simulink library "PMSM_Library"  (R2023a)
settings: Solver=VariableStepAuto  StartTime=0.0  StopTime=10.0  RelTol=1e-3  EnableMultiTasking=on
settings Model: Creator=michaelsun  LastModifiedBy=洲
settings SolverCC: AlgebraicLoopSolver=TrustRegion
settings DataIOCC: LimitDataPoints=on
settings OptimizationCC: LifeSpan=inf
settings DebuggingCC: UnconnectedInputMsg=warning  UnconnectedOutputMsg=warning  UnconnectedLineMsg=warning  AllowSymbolicDim=off  SFUnexpectedBacktrackingDiag=warning  SFNoUnconditionalDefaultTransitionDiag=warning  SFExecutionAtInitializationDiag=none  ArithmeticOperatorsInVariantConditions=warning
settings ModelReferenceCC: EnableRefExpFcnMdlSchedulingChecks=on  PropagateSignalLabelsOutOfModel=off
settings SFSimCC: SimUseLocalCustomCode=off  CustomCodeUndefinedFunction=UseInterfaceOnly
settings RTWCC: RTWUseLocalCustomCode=off  DLArmComputeVersion=19.05
settings CodeAppCC: StateflowObjectComments=on
settings GRTTargetCC: TargetLangStandard=C89/C90 (ANSI)
settings ConfigComp: CovMetricSettings=dw  CovSaveCumulativeToWorkspaceVar=on  CovSaveSingleToWorkspaceVar=on  CovExternalEMLEnable=off

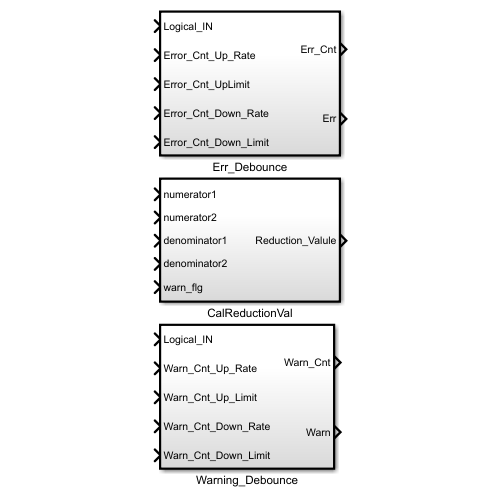
[thumbnail: Simulink's stored preview of the top-level diagram]
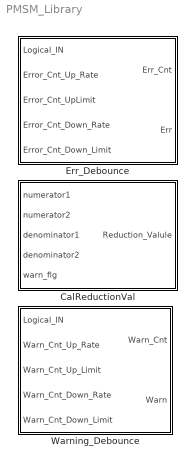
== system PMSM_Library ==
  CalReductionVal : Subsystem  TreatAsAtomicUnit=on  RTWFcnName=CalReductionVal  RTWFileName=CalReductionVal
      settings: RTWSystemCode=Inline  RTWFcnNameOpts=User specified  RTWFileNameOpts=User specified
  Err_Debounce : Subsystem  TreatAsAtomicUnit=on  RTWFcnName=Err_Debounce  RTWFileName=Err_Debounce
      settings: RTWSystemCode=Inline  RTWFcnNameOpts=User specified  RTWFileNameOpts=User specified
  Warning_Debounce : Subsystem  TreatAsAtomicUnit=on  RTWFcnName=Warning_Debounce  RTWFileName=Warning_Debounce
      settings: RTWSystemCode=Inline  RTWFcnNameOpts=User specified  RTWFileNameOpts=User specified

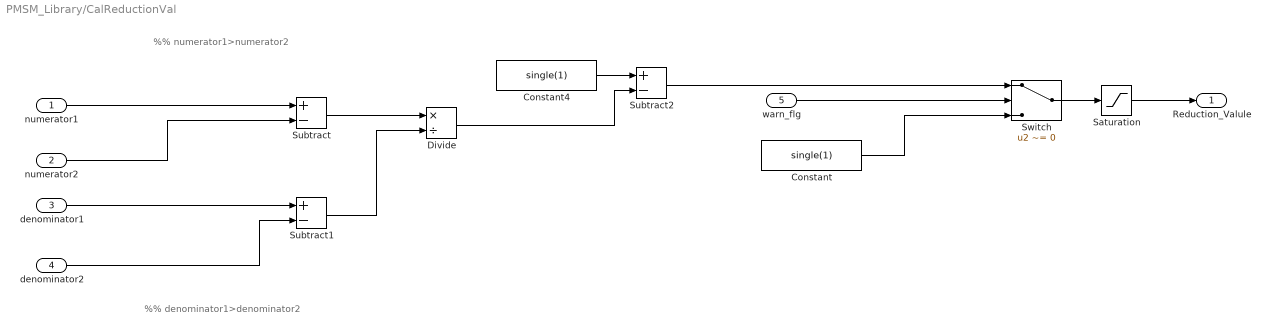
== system PMSM_Library/CalReductionVal ==
  note: %% numerator1>numerator2
  note: %% denominator1>denominator2
  numerator1 : Inport
  numerator2 : Inport  Port=2
  denominator1 : Inport  Port=3
  denominator2 : Inport  Port=4
  warn_flg : Inport  Port=5
  Constant : Constant  Value=single(1)
  Constant4 : Constant  Value=single(1)
  Divide : Product  Inputs=*/
  Saturation : Saturate  UpperLimit=1.0  LowerLimit=0.0
  Subtract : Sum  Inputs=+-
  Subtract1 : Sum  Inputs=+-
  Subtract2 : Sum  Inputs=+-
  Switch : Switch  Criteria=u2 ~= 0  SaturateOnIntegerOverflow=off  InputSameDT=off
  Reduction_Valule : Outport
  wires:
  Saturation/1 -> Reduction_Valule/1
  numerator2/1 -> Subtract/2
  denominator1/1 -> Subtract1/1
  denominator2/1 -> Subtract1/2
  Constant4/1 -> Subtract2/1
  Constant/1 -> Switch/3
  warn_flg/1 -> Switch/2
  Switch/1 -> Saturation/1
  Subtract2/1 -> Switch/1
  Divide/1 -> Subtract2/2
  Subtract1/1 -> Divide/2
  Subtract/1 -> Divide/1
  numerator1/1 -> Subtract/1

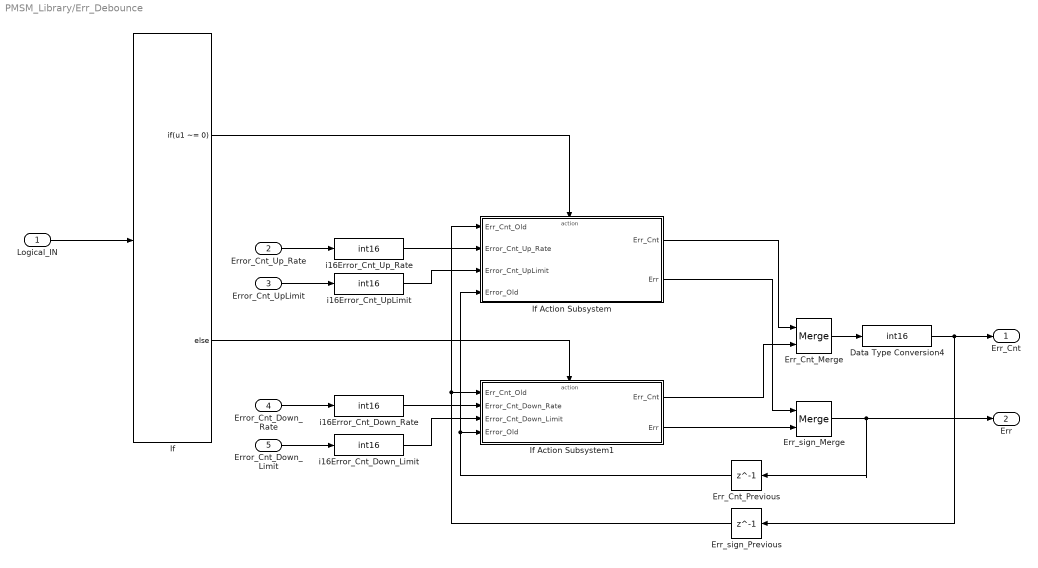
== system PMSM_Library/Err_Debounce ==
  Logical_IN : Inport
  Error_Cnt_Up_Rate : Inport  Port=2
  Error_Cnt_UpLimit : Inport  Port=3
  Error_Cnt_Down_Rate : Inport  Port=4
  Error_Cnt_Down_Limit : Inport  Port=5
  Data Type Conversion4 : DataTypeConversion  OutDataTypeStr=int16  SaturateOnIntegerOverflow=off  RndMeth=Floor
  Err_Cnt_Merge : Merge
  Err_Cnt_Previous : Delay  DelayLength=1  InitialCondition=boolean(0)
  Err_sign_Merge : Merge
  Err_sign_Previous : Delay  DelayLength=1
  If : If  IfExpression=u1 ~= 0
  If Action Subsystem : Subsystem  TreatAsAtomicUnit=on
  If Action Subsystem1 : Subsystem  TreatAsAtomicUnit=on
  i16Error_Cnt_Down_Limit : DataTypeConversion  OutDataTypeStr=int16  SaturateOnIntegerOverflow=off  RndMeth=Floor
  i16Error_Cnt_Down_Rate : DataTypeConversion  OutDataTypeStr=int16  SaturateOnIntegerOverflow=off  RndMeth=Floor
  i16Error_Cnt_UpLimit : DataTypeConversion  OutDataTypeStr=int16  SaturateOnIntegerOverflow=off  RndMeth=Floor
  i16Error_Cnt_Up_Rate : DataTypeConversion  OutDataTypeStr=int16  SaturateOnIntegerOverflow=off  RndMeth=Floor
  Err_Cnt : Outport
  Err : Outport  Port=2
  wires:
  Data Type Conversion4/1 -> Err_sign_Previous/1, Err_Cnt/1
  i16Error_Cnt_Up_Rate/1 -> If Action Subsystem/2(Error_Cnt_Up_Rate)
  i16Error_Cnt_UpLimit/1 -> If Action Subsystem/3(Error_Cnt_UpLimit)
  i16Error_Cnt_Down_Rate/1 -> If Action Subsystem1/2(Error_Cnt_Down_Rate)
  i16Error_Cnt_Down_Limit/1 -> If Action Subsystem1/3(Error_Cnt_Down_Limit)
  Err_Cnt_Previous/1 -> If Action Subsystem/4(Error_Old), If Action Subsystem1/4(Error_Old)
  Err_sign_Merge/1 -> Err/1, Err_Cnt_Previous/1
  If Action Subsystem/2(Err) -> Err_sign_Merge/1
  If Action Subsystem1/2(Err) -> Err_sign_Merge/2
  Error_Cnt_Down_Limit/1 -> i16Error_Cnt_Down_Limit/1
  Error_Cnt_Up_Rate/1 -> i16Error_Cnt_Up_Rate/1
  Error_Cnt_Down_Rate/1 -> i16Error_Cnt_Down_Rate/1
  Logical_IN/1 -> If/1
  Error_Cnt_UpLimit/1 -> i16Error_Cnt_UpLimit/1
  If Action Subsystem1/1(Err_Cnt) -> Err_Cnt_Merge/2
  If Action Subsystem/1(Err_Cnt) -> Err_Cnt_Merge/1
  If/2 -> If Action Subsystem1/Action
  If/1 -> If Action Subsystem/Action
  Err_sign_Previous/1 -> If Action Subsystem1/1(Err_Cnt_Old), If Action Subsystem/1(Err_Cnt_Old)
  Err_Cnt_Merge/1 -> Data Type Conversion4/1

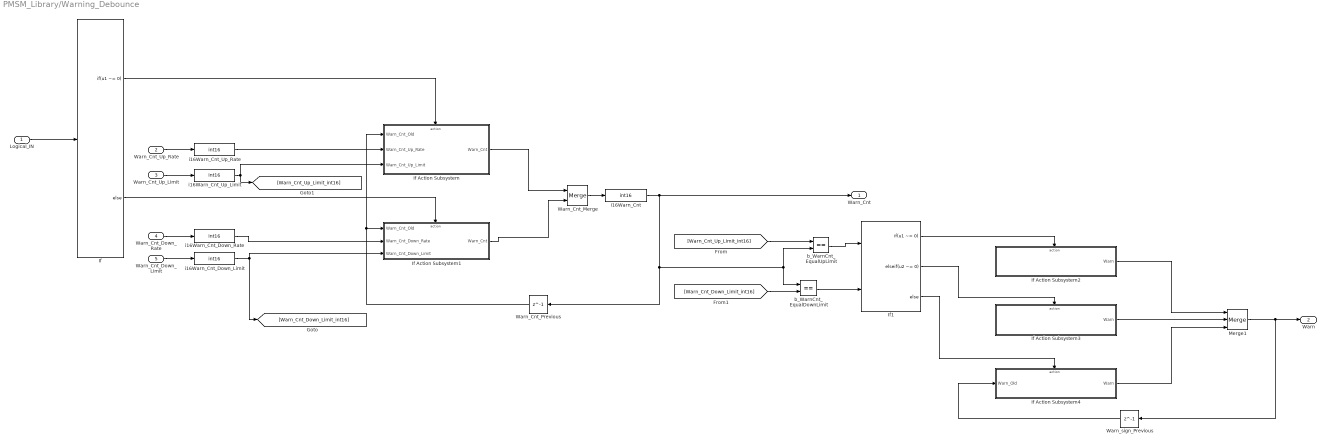
== system PMSM_Library/Warning_Debounce ==
  Logical_IN : Inport
  Warn_Cnt_Up_Rate : Inport  Port=2
  Warn_Cnt_Up_Limit : Inport  Port=3
  Warn_Cnt_Down_Rate : Inport  Port=4
  Warn_Cnt_Down_Limit : Inport  Port=5
  If : If  IfExpression=u1 ~= 0
  If Action Subsystem : Subsystem  TreatAsAtomicUnit=on
  If Action Subsystem1 : Subsystem  TreatAsAtomicUnit=on
  If Action Subsystem2 : Subsystem  TreatAsAtomicUnit=on
  If Action Subsystem3 : Subsystem  TreatAsAtomicUnit=on
  If Action Subsystem4 : Subsystem  TreatAsAtomicUnit=on
  If1 : If  NumInputs=2  IfExpression=u1 ~= 0  ElseIfExpressions=u2 ~= 0
  Merge1 : Merge  Inputs=3
  Warn_Cnt_Merge : Merge
  Warn_Cnt_Previous : Delay  DelayLength=1
  Warn_sign_Previous : Delay  DelayLength=1
  b_WarnCnt_EqualDownLimit : RelationalOperator  Operator===  OutDataTypeStr=boolean  InputSameDT=off
  b_WarnCnt_EqualUpLimit : RelationalOperator  Operator===  OutDataTypeStr=boolean  InputSameDT=off
  i16Warn_Cnt : DataTypeConversion  OutDataTypeStr=int16  SaturateOnIntegerOverflow=off  RndMeth=Floor
  i16Warn_Cnt_Down_Limit : DataTypeConversion  OutDataTypeStr=int16  SaturateOnIntegerOverflow=off  RndMeth=Floor
  i16Warn_Cnt_Down_Rate : DataTypeConversion  OutDataTypeStr=int16  SaturateOnIntegerOverflow=off  RndMeth=Floor
  i16Warn_Cnt_Up_Limit : DataTypeConversion  OutDataTypeStr=int16  SaturateOnIntegerOverflow=off  RndMeth=Floor
  i16Warn_Cnt_Up_Rate : DataTypeConversion  OutDataTypeStr=int16  SaturateOnIntegerOverflow=off  RndMeth=Floor
  Warn_Cnt : Outport
  Warn : Outport  Port=2
  wires:
  Warn_sign_Previous/1 -> If Action Subsystem4/1(Warn_Old)
  Merge1/1 -> Warn/1, Warn_sign_Previous/1
  If Action Subsystem4/1(Warn) -> Merge1/3
  If Action Subsystem2/1(Warn) -> Merge1/1
  If Action Subsystem3/1(Warn) -> Merge1/2
  If1/3 -> If Action Subsystem4/Action
  If1/2 -> If Action Subsystem3/Action
  If1/1 -> If Action Subsystem2/Action
  b_WarnCnt_EqualDownLimit/1 -> If1/2
  b_WarnCnt_EqualUpLimit/1 -> If1/1
  [Warn_Cnt_Down_Limit_int16] -> b_WarnCnt_EqualDownLimit/2
  [Warn_Cnt_Up_Limit_int16] -> b_WarnCnt_EqualUpLimit/1
  Warn_Cnt_Merge/1 -> i16Warn_Cnt/1
  Warn_Cnt_Previous/1 -> If Action Subsystem/1(Warn_Cnt_Old), If Action Subsystem1/1(Warn_Cnt_Old)
  If/1 -> If Action Subsystem/Action
  If/2 -> If Action Subsystem1/Action
  If Action Subsystem/1(Warn_Cnt) -> Warn_Cnt_Merge/1
  If Action Subsystem1/1(Warn_Cnt) -> Warn_Cnt_Merge/2
  Warn_Cnt_Up_Limit/1 -> i16Warn_Cnt_Up_Limit/1
  Logical_IN/1 -> If/1
  Warn_Cnt_Down_Rate/1 -> i16Warn_Cnt_Down_Rate/1
  Warn_Cnt_Up_Rate/1 -> i16Warn_Cnt_Up_Rate/1
  Warn_Cnt_Down_Limit/1 -> i16Warn_Cnt_Down_Limit/1
  i16Warn_Cnt_Down_Limit/1 -> If Action Subsystem1/3(Warn_Cnt_Down_Limit), [Warn_Cnt_Down_Limit_int16]
  i16Warn_Cnt_Down_Rate/1 -> If Action Subsystem1/2(Warn_Cnt_Down_Rate)
  i16Warn_Cnt_Up_Limit/1 -> [Warn_Cnt_Up_Limit_int16], If Action Subsystem/3(Warn_Cnt_Up_Limit)
  i16Warn_Cnt_Up_Rate/1 -> If Action Subsystem/2(Warn_Cnt_Up_Rate)
  i16Warn_Cnt/1 -> Warn_Cnt/1, Warn_Cnt_Previous/1, b_WarnCnt_EqualUpLimit/2, b_WarnCnt_EqualDownLimit/1

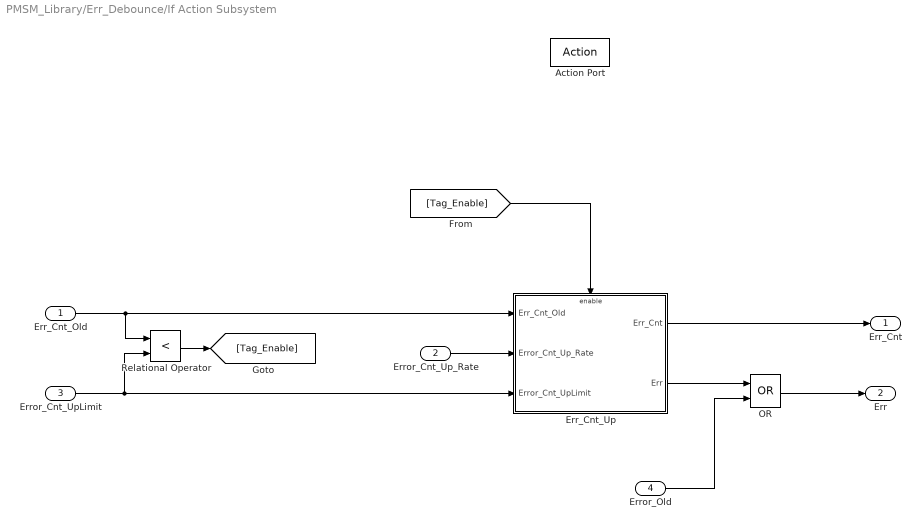
== system PMSM_Library/Err_Debounce/If Action Subsystem ==
  Err_Cnt_Old : Inport
  Error_Cnt_Up_Rate : Inport  Port=2
  Error_Cnt_UpLimit : Inport  Port=3
  Error_Old : Inport  Port=4
  Action Port : ActionPort
  Err_Cnt_Up : Subsystem  RTWFcnName=Err_Cnt_Up
      settings: RTWSystemCode=Inline  RTWFcnNameOpts=User specified
  OR : Logic  Operator=OR  AllPortsSameDT=off  OutDataTypeStr=boolean
  Relational Operator : RelationalOperator  Operator=<  OutDataTypeStr=boolean  InputSameDT=off
  Err_Cnt : Outport
  Err : Outport  Port=2
  wires:
  [Tag_Enable] -> Err_Cnt_Up/Enable
  Relational Operator/1 -> [Tag_Enable]
  Err_Cnt_Up/2(Err) -> OR/1
  Err_Cnt_Up/1(Err_Cnt) -> Err_Cnt/1
  Error_Cnt_UpLimit/1 -> Relational Operator/2, Err_Cnt_Up/3(Error_Cnt_UpLimit)
  Error_Cnt_Up_Rate/1 -> Err_Cnt_Up/2(Error_Cnt_Up_Rate)
  Err_Cnt_Old/1 -> Err_Cnt_Up/1(Err_Cnt_Old), Relational Operator/1
  Error_Old/1 -> OR/2
  OR/1 -> Err/1

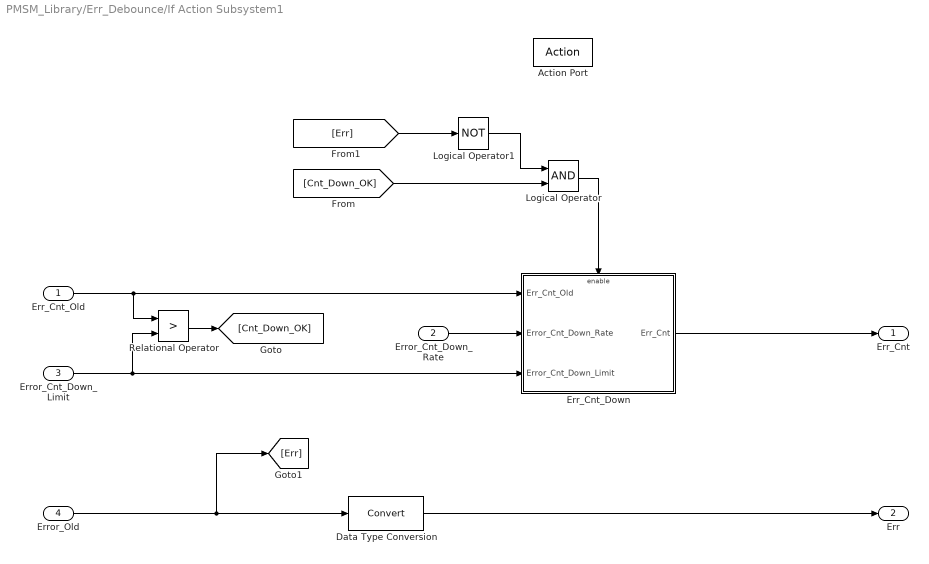
== system PMSM_Library/Err_Debounce/If Action Subsystem1 ==
  Err_Cnt_Old : Inport
  Error_Cnt_Down_Rate : Inport  Port=2
  Error_Cnt_Down_Limit : Inport  Port=3
  Error_Old : Inport  Port=4
  Action Port : ActionPort
  Data Type Conversion : DataTypeConversion  SaturateOnIntegerOverflow=off  RndMeth=Floor
  Err_Cnt_Down : Subsystem  RTWFcnName=Err_Cnt_Down
      settings: RTWSystemCode=Inline  RTWFcnNameOpts=User specified
  Logical Operator : Logic  AllPortsSameDT=off  OutDataTypeStr=boolean
  Logical Operator1 : Logic  Operator=NOT  AllPortsSameDT=off  OutDataTypeStr=boolean
  Relational Operator : RelationalOperator  Operator=>  OutDataTypeStr=boolean  InputSameDT=off
  Err_Cnt : Outport
  Err : Outport  Port=2
  wires:
  Data Type Conversion/1 -> Err/1
  Error_Old/1 -> Data Type Conversion/1, [Err]
  Logical Operator1/1 -> Logical Operator/1
  [Err] -> Logical Operator1/1
  Logical Operator/1 -> Err_Cnt_Down/Enable
  [Cnt_Down_OK] -> Logical Operator/2
  Error_Cnt_Down_Rate/1 -> Err_Cnt_Down/2(Error_Cnt_Down_Rate)
  Relational Operator/1 -> [Cnt_Down_OK]
  Err_Cnt_Down/1(Err_Cnt) -> Err_Cnt/1
  Error_Cnt_Down_Limit/1 -> Relational Operator/2, Err_Cnt_Down/3(Error_Cnt_Down_Limit)
  Err_Cnt_Old/1 -> Err_Cnt_Down/1(Err_Cnt_Old), Relational Operator/1

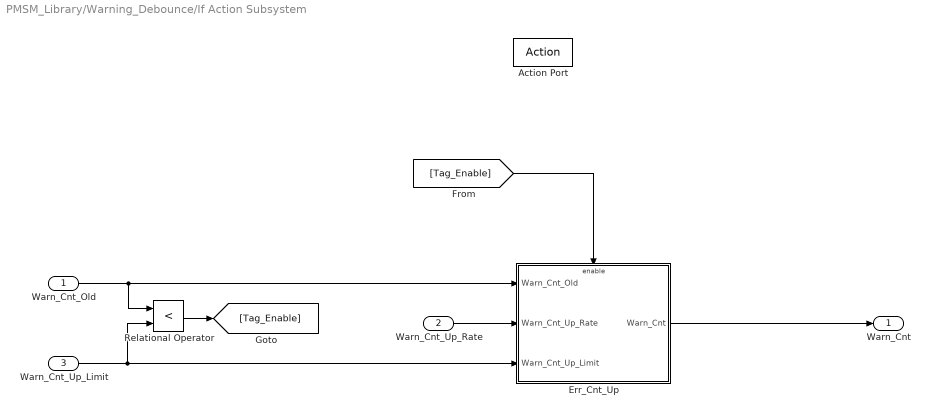
== system PMSM_Library/Warning_Debounce/If Action Subsystem ==
  Warn_Cnt_Old : Inport
  Warn_Cnt_Up_Rate : Inport  Port=2
  Warn_Cnt_Up_Limit : Inport  Port=3
  Action Port : ActionPort
  Err_Cnt_Up : Subsystem
  Relational Operator : RelationalOperator  Operator=<  OutDataTypeStr=boolean  InputSameDT=off
  Warn_Cnt : Outport
  wires:
  Warn_Cnt_Old/1 -> Relational Operator/1, Err_Cnt_Up/1(Warn_Cnt_Old)
  Warn_Cnt_Up_Rate/1 -> Err_Cnt_Up/2(Warn_Cnt_Up_Rate)
  Warn_Cnt_Up_Limit/1 -> Err_Cnt_Up/3(Warn_Cnt_Up_Limit), Relational Operator/2
  Err_Cnt_Up/1(Warn_Cnt) -> Warn_Cnt/1
  Relational Operator/1 -> [Tag_Enable]
  [Tag_Enable] -> Err_Cnt_Up/Enable

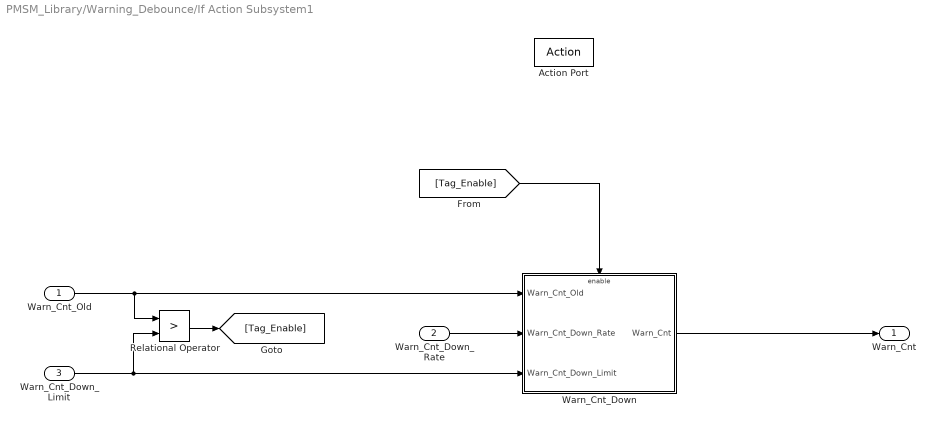
== system PMSM_Library/Warning_Debounce/If Action Subsystem1 ==
  Warn_Cnt_Old : Inport
  Warn_Cnt_Down_Rate : Inport  Port=2
  Warn_Cnt_Down_Limit : Inport  Port=3
  Action Port : ActionPort
  Relational Operator : RelationalOperator  Operator=>  OutDataTypeStr=boolean  InputSameDT=off
  Warn_Cnt_Down : Subsystem
  Warn_Cnt : Outport
  wires:
  Warn_Cnt_Old/1 -> Relational Operator/1, Warn_Cnt_Down/1(Warn_Cnt_Old)
  Warn_Cnt_Down_Limit/1 -> Warn_Cnt_Down/3(Warn_Cnt_Down_Limit), Relational Operator/2
  Warn_Cnt_Down/1(Warn_Cnt) -> Warn_Cnt/1
  Relational Operator/1 -> [Tag_Enable]
  [Tag_Enable] -> Warn_Cnt_Down/Enable
  Warn_Cnt_Down_Rate/1 -> Warn_Cnt_Down/2(Warn_Cnt_Down_Rate)

== system PMSM_Library/Warning_Debounce/If Action Subsystem2 ==
  Action Port : ActionPort
  Constant : Constant  Value=boolean(1)
  Warn : Outport
  wires:
  Constant/1 -> Warn/1

== system PMSM_Library/Warning_Debounce/If Action Subsystem3 ==
  Action Port : ActionPort
  Constant : Constant  Value=boolean(0)
  Warn : Outport
  wires:
  Constant/1 -> Warn/1

== system PMSM_Library/Warning_Debounce/If Action Subsystem4 ==
  Warn_Old : Inport
  Action Port : ActionPort
  Warn : Outport
  wires:
  Warn_Old/1 -> Warn/1

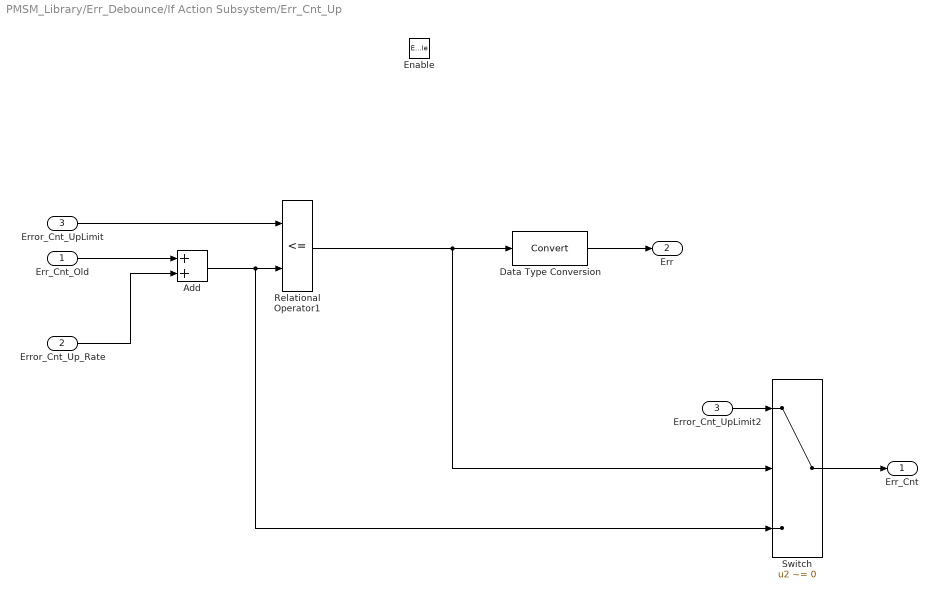
== system PMSM_Library/Err_Debounce/If Action Subsystem/Err_Cnt_Up ==
  Err_Cnt_Old : Inport
  Error_Cnt_Up_Rate : Inport  Port=2
  Error_Cnt_UpLimit : Inport  Port=3
  Enable : EnablePort
  Add : Sum
  Data Type Conversion : DataTypeConversion  SaturateOnIntegerOverflow=off  RndMeth=Floor
  Error_Cnt_UpLimit2 : InportShadow  Port=3
  Relational Operator1 : RelationalOperator  Operator=<=  OutDataTypeStr=boolean  ZeroCross=off  InputSameDT=off
  Switch : Switch  Criteria=u2 ~= 0  SaturateOnIntegerOverflow=off  InputSameDT=off
  Err_Cnt : Outport
  Err : Outport  Port=2
  wires:
  Data Type Conversion/1 -> Err/1
  Relational Operator1/1 -> Data Type Conversion/1, Switch/2
  Error_Cnt_UpLimit2/1 -> Switch/1
  Switch/1 -> Err_Cnt/1
  Error_Cnt_UpLimit/1 -> Relational Operator1/1
  Error_Cnt_Up_Rate/1 -> Add/2
  Err_Cnt_Old/1 -> Add/1
  Add/1 -> Switch/3, Relational Operator1/2

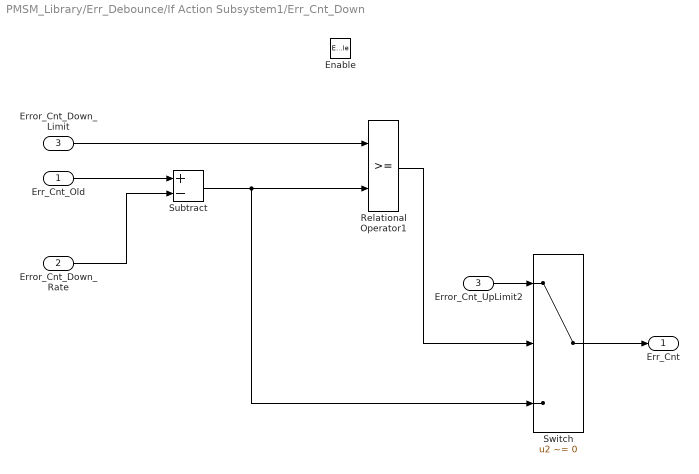
== system PMSM_Library/Err_Debounce/If Action Subsystem1/Err_Cnt_Down ==
  Err_Cnt_Old : Inport
  Error_Cnt_Down_Rate : Inport  Port=2
  Error_Cnt_Down_Limit : Inport  Port=3
  Enable : EnablePort
  Error_Cnt_UpLimit2 : InportShadow  Port=3
  Relational Operator1 : RelationalOperator  OutDataTypeStr=boolean  InputSameDT=off
  Subtract : Sum  Inputs=+-
  Switch : Switch  Criteria=u2 ~= 0  SaturateOnIntegerOverflow=off  InputSameDT=off
  Err_Cnt : Outport
  wires:
  Error_Cnt_UpLimit2/1 -> Switch/1
  Switch/1 -> Err_Cnt/1
  Error_Cnt_Down_Limit/1 -> Relational Operator1/1
  Relational Operator1/1 -> Switch/2
  Error_Cnt_Down_Rate/1 -> Subtract/2
  Err_Cnt_Old/1 -> Subtract/1
  Subtract/1 -> Switch/3, Relational Operator1/2

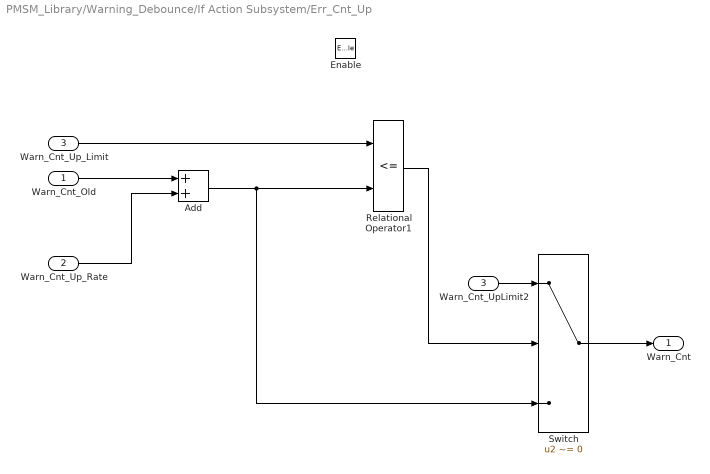
== system PMSM_Library/Warning_Debounce/If Action Subsystem/Err_Cnt_Up ==
  Warn_Cnt_Old : Inport
  Warn_Cnt_Up_Rate : Inport  Port=2
  Warn_Cnt_Up_Limit : Inport  Port=3
  Enable : EnablePort
  Add : Sum
  Relational Operator1 : RelationalOperator  Operator=<=  OutDataTypeStr=boolean  InputSameDT=off
  Switch : Switch  Criteria=u2 ~= 0  SaturateOnIntegerOverflow=off  InputSameDT=off
  Warn_Cnt_UpLimit2 : InportShadow  Port=3
  Warn_Cnt : Outport
  wires:
  Add/1 -> Relational Operator1/2, Switch/3
  Warn_Cnt_Old/1 -> Add/1
  Warn_Cnt_Up_Rate/1 -> Add/2
  Relational Operator1/1 -> Switch/2
  Warn_Cnt_Up_Limit/1 -> Relational Operator1/1
  Switch/1 -> Warn_Cnt/1
  Warn_Cnt_UpLimit2/1 -> Switch/1

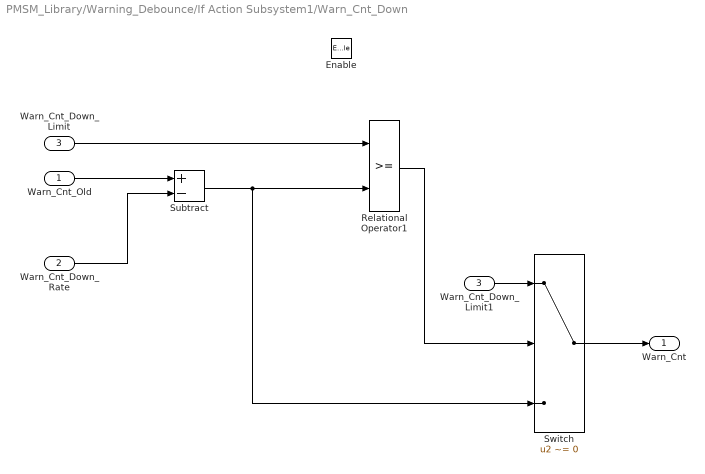
== system PMSM_Library/Warning_Debounce/If Action Subsystem1/Warn_Cnt_Down ==
  Warn_Cnt_Old : Inport
  Warn_Cnt_Down_Rate : Inport  Port=2
  Warn_Cnt_Down_Limit : Inport  Port=3
  Enable : EnablePort
  Relational Operator1 : RelationalOperator  OutDataTypeStr=boolean  InputSameDT=off
  Subtract : Sum  Inputs=+-
  Switch : Switch  Criteria=u2 ~= 0  SaturateOnIntegerOverflow=off  InputSameDT=off
  Warn_Cnt_Down_Limit1 : InportShadow  Port=3
  Warn_Cnt : Outport
  wires:
  Relational Operator1/1 -> Switch/2
  Subtract/1 -> Relational Operator1/2, Switch/3
  Warn_Cnt_Old/1 -> Subtract/1
  Warn_Cnt_Down_Rate/1 -> Subtract/2
  Warn_Cnt_Down_Limit/1 -> Relational Operator1/1
  Switch/1 -> Warn_Cnt/1
  Warn_Cnt_Down_Limit1/1 -> Switch/1
